simulink model "quantized_bpf_test"  (R2021b)
settings: Solver=VariableStepAuto  StartTime=0.0  StopTime=10.0  RelTol=1e-3
libraries: dspsnks4 x1, dsparch4 x1, dspvision x1
settings Model: Creator=caccolillo  LastModifiedBy=caccolillo
settings DebuggingCC: SignalRangeChecking=warning

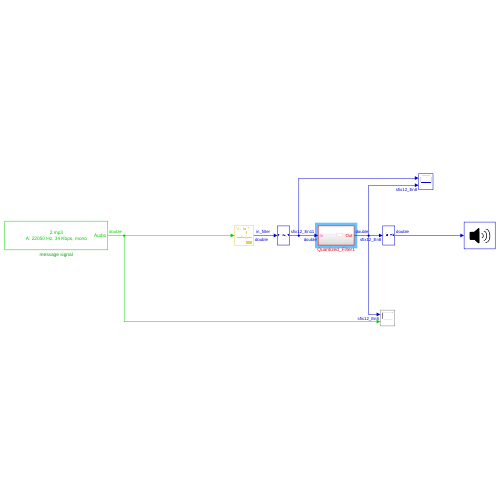
[thumbnail: Simulink's stored preview of the top-level diagram]
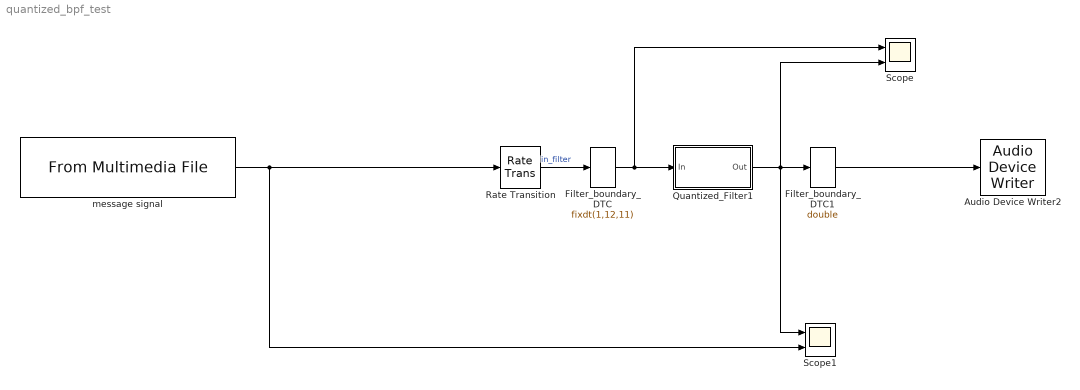
== system quantized_bpf_test ==
  Audio Device Writer2 : dspsnks4/Audio Device Writer  Driver=ALSA  Device=Default  InheritSampleRate=on  SampleRate=44100  BitDepth=32-bit float  BufferSize=4096  NumBuffers=10  DefaultOutputChannelMapping=on  OutputChannelMapping=1:2  OutputNumUnderrunSamples=off  DriverIdx=8  DeviceWarnFlag=''
  Filter_boundary_DTC : DataTypeConversion  OutDataTypeStr=fixdt(1,12,11)  SaturateOnIntegerOverflow=on  RndMeth=Zero
  Filter_boundary_DTC1 : DataTypeConversion  OutDataTypeStr=double  SaturateOnIntegerOverflow=on  RndMeth=Zero
  Quantized_Filter1 : Subsystem  Tag=BlockMethodSubSystem
  Rate Transition : RateTransition  Deterministic=off  OutPortSampleTime=1/8000
  Scope : Scope  NumInputPorts=2
  Scope1 : Scope  NumInputPorts=2
  message signal : dspvision/From Multimedia File  inputFilename=/home/caccolillo/Downloads/test_filter_colin/audio/2.mp3  readRange=[1 Inf]  loop=on  numPlays=inf  outputStreams=Audio only  videoDataType=single  audioDataType=double  inheritSampleTime=on  userDefinedSampleTime=1/30  noAudioOutput=off  isIntensityVideo=off  fourcc=RGB  colorVideoFormat=Separate color signals  outputEOF=off  dataOrg=Column-major  audioFrameSize=1  computeAudioFrameSize=off  outSamplingMode=Frame based
  wires:
  message signal/1 -> Rate Transition/1, Scope1/2
  Rate Transition/1 -> Filter_boundary_DTC/1  "in_filter"
  Filter_boundary_DTC/1 -> Quantized_Filter1/1(In), Scope/1
  Quantized_Filter1/1(Out) -> Scope/2, Scope1/1, Filter_boundary_DTC1/1
  Filter_boundary_DTC1/1 -> Audio Device Writer2/1

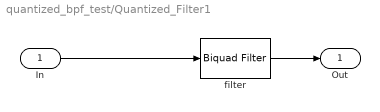
== system quantized_bpf_test/Quantized_Filter1 ==
  In : Inport
  filter : dsparch4/Biquad Filter  FilterSource=Dialog parameters  CoeffSource=Specify via dialog  FilterObject=BQF  IIRFiltStruct=Direct form II  BiQuadCoeffs=[1 0 -1 1 1.65742528830292724 0.815897372432069612;1 0 -1 1 -1.85998922851952742 0.901702779731603621;1 0 -1 1 -1.70469105875488869 0.744422984879922978;1 0 -1 1 1.41335332460150043 0.553995092737038175;1 0 -1 1 -1.61545832429382541 0.654784747265885092;1 0 -1 1 1.28646306613610628 0.420394826751919415]  ScaleValues=[0.885889217627322534;0.885889217627322534;0.799139044168098667;0.799139044168098667;0.759352137722818288;0.759352137722818288;1]  IC=0  ICnum=0  ICden=0  a0Flag=Warning  optimizeScaleValues=on  ScaleValueMode=Specify via input port (g)  InputProcessing=Columns as channels (frame based)  roundingMode=Convergent  overflowMode=on  stageInputMode=Binary point scaling  stageInputWordLength=12  stageInputFracLength=7  stageOutputMode=Binary point scaling  stageOutputWordLength=12  stageOutputFracLength=8  firstCoeffMode=Binary point scaling  firstCoeffWordLength=12  firstCoeffFracLength=10  scaleValueFracLength=11  prodOutputMode=Binary point scaling  prodOutputWordLength=60  prodOutputFracLength=42  denProdOutputFracLength=22  accumMode=Binary point scaling  accumWordLength=60  accumFracLength=42  denAccumFracLength=22  memoryMode=Binary point scaling  memoryWordLength=60  memoryFracLength=42  secondMemoryFracLength=15  outputMode=Binary point scaling  outputWordLength=12  outputFracLength=8
  Out : Outport
  wires:
  filter/1 -> Out/1
  In/1 -> filter/1
